simulink model "Sim_System"  (R2021a)
settings: Solver=VariableStepAuto  StartTime=0.0  StopTime=15  RelTol=1e-3
values from neighbouring files (symbols this model uses):
  f_0 = [ f_10; 1 - f_10 ]    [simulink_params.m]
  nu = [ 0.1 0.7 ]    [dilution_model.m]    (also in simulink_params.m = min(max(1 - chi/alpha, zeros(2,1)), ones(2,1)))
  s = [ 0.6 0.7 ]    [dilution_model.m]    (also in simulink_params.m = s0 - m*chi)
undefined symbols (not defined in the file or in its folder): DiscIntNeverNeededParam
settings Model: Creator=Ben  LastModifiedBy=Ben

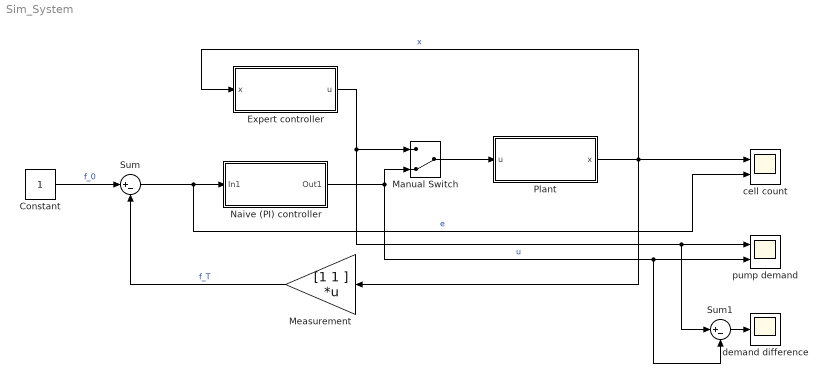
== system Sim_System ==
  Constant : Constant
  Expert controller : Subsystem
  Manual Switch : ManualSwitch  CurrentSetting=0
  Measurement : Gain  Gain=[1 1 ]  Multiplication=Matrix(K*u)
  Naive (PI) controller : Subsystem
  Plant : Subsystem
  Sum : Sum  Inputs=|+-
  Sum1 : Sum  Inputs=|+-
  cell count : Scope  NumInputPorts=2
  demand difference : Scope
  pump demand : Scope  NumInputPorts=2
  wires:
  Constant/1 -> Sum/1  "f_0"
  Measurement/1 -> Sum/2  "f_T"
  Sum/1 -> cell count/2, Naive (PI) controller/1(In1)  "e"
  Naive (PI) controller/1(Out1) -> pump demand/2, Sum1/2, Manual Switch/2  "u"
  Plant/1(x) -> Measurement/1, cell count/1, Expert controller/1(x)  "x"
  Manual Switch/1 -> Plant/1(u)
  Expert controller/1(u) -> Sum1/1, pump demand/1, Manual Switch/1
  Sum1/1 -> demand difference/1

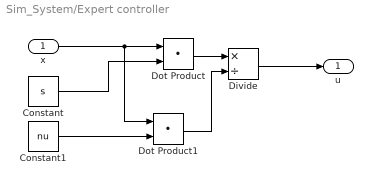
== system Sim_System/Expert controller ==
  x : Inport
  Constant : Constant  Value=s
  Constant1 : Constant  Value=nu
  Divide : Product  Inputs=*/
  Dot Product : DotProduct  InputSameDT=on  OutDataTypeStr=Inherit: Inherit via internal rule
  Dot Product1 : DotProduct  InputSameDT=on  OutDataTypeStr=Inherit: Inherit via internal rule
  u : Outport
  wires:
  x/1 -> Dot Product1/1, Dot Product/1
  Dot Product/1 -> Divide/1
  Constant/1 -> Dot Product/2
  Constant1/1 -> Dot Product1/2
  Dot Product1/1 -> Divide/2
  Divide/1 -> u/1

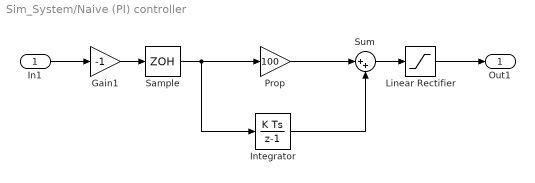
== system Sim_System/Naive (PI) controller ==
  In1 : Inport
  Gain1 : Gain  Gain=-1
  Integrator : DiscreteIntegrator  gainval=30  SampleTime=-1  ICPrevOutput=DiscIntNeverNeededParam  ICPrevScaledInput=DiscIntNeverNeededParam
  Linear Rectifier : Saturate  UpperLimit=inf  LowerLimit=0
  Prop : Gain  Gain=100
  Sample : ZeroOrderHold  SampleTime=1e-2
  Sum : Sum  Inputs=|++
  Out1 : Outport
  wires:
  Sample/1 -> Integrator/1, Prop/1
  Prop/1 -> Sum/1
  Integrator/1 -> Sum/2
  Sum/1 -> Linear Rectifier/1
  Linear Rectifier/1 -> Out1/1
  In1/1 -> Gain1/1
  Gain1/1 -> Sample/1

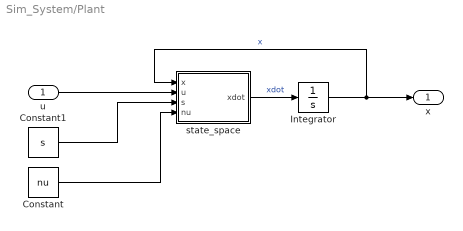
== system Sim_System/Plant ==
  u : Inport
  Constant : Constant  Value=nu
  Constant1 : Constant  Value=s
  Integrator : Integrator  InitialCondition=f_0
  state_space : MATLAB Function  TreatAsAtomicUnit=on
  x : Outport
  wires:
  Constant/1 -> state_space/4(nu)
  u/1 -> state_space/2(u)
  Constant1/1 -> state_space/3(s)
  Integrator/1 -> state_space/1(x), x/1  "x"
  state_space/1(xdot) -> Integrator/1  "xdot"

== matlab function Sim_System/Plant/state_space ==
  data: x input; u input; xdot output; s input; nu input
function xdot = ss(x, u, s, nu)

A = diag(s - nu*u);

xdot = A*x;
